simulink model "position_control"  (R2022a)
settings: Solver=ode1  StartTime=0.0  StopTime=inf  FixedStep=0.001  RelTol=1e-3
undefined symbols (not defined in the file or in its folder): a, b, k1, k2, kd2, kd4, kp2, kp4
libraries: arduinolib x19, arduinosensorlib x6, simulink_extras x2, visionfilter x1, eeLuenbergerObserver x1
settings Model: SimulationMode=external  ExtModeTrigDuration=2  Creator=DCLab  LastModifiedBy=LabPC
settings SolverCC: AllowMultiTaskInputOutput=on
settings OptimizationCC: EnhancedBackFolding=on  PassReuseOutputArgsAs=Individual arguments  ZeroExternalMemoryAtStartup=off  ZeroInternalMemoryAtStartup=off  MaxStackSize=64  OptimizeBlockOrder=speed  DifferentSizesBufferReuse=on  OptimizationCustomize=off  EfficientTunableParamExpr=on
settings DebuggingCC: ParameterTunabilityLossMsg=error  UnconnectedInputMsg=warning  UnconnectedOutputMsg=warning  UnconnectedLineMsg=warning
settings HardwareCC: ProdBitPerPointer=32  ProdBitPerSizeT=32  ProdBitPerPtrDiffT=32  ProdLargestAtomicInteger=Long  ProdLargestAtomicFloat=Double  ProdWordSize=32  ProdHWDeviceType=ARM Compatible->ARM Cortex
settings SFSimCC: MATLABDynamicMemAlloc=off  SimTargetLang=C++
settings RTWCC: SystemTargetFile=ert.tlc  HardwareBoard=Arduino Due  TemplateMakefile=ert_default_tmf  Toolchain=Arduino ARM  BuildConfiguration=Faster Runs  DLArmComputeVersion=19.05
settings CodeAppCC: ForceParamTrailComments=on  IgnoreCustomStorageClasses=off  OperatorAnnotations=on  SimulinkDataObjDesc=on  SFDataObjDesc=on  InsertBlockDesc=on
settings ERTTargetCC: SupportContinuousTime=on  SupportVariableSizeSignals=on  ExtMode=on  ExtModeTransport=3  ExtModeStaticAlloc=on  ExtModeStaticAllocSize=24576  ExtModeMexFile=ext_xcp  ExtModeMexArgs=0 3 115200  ExtModeIntrfLevel=Level2 - Open

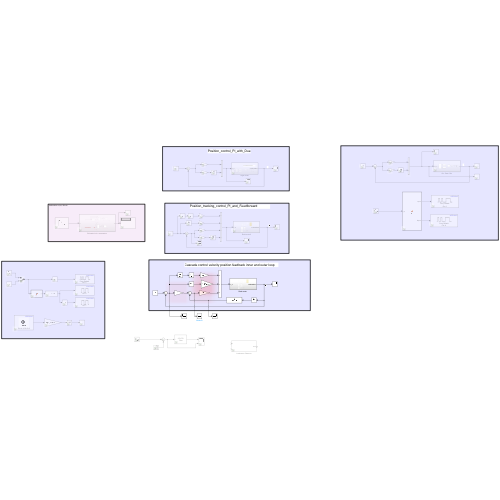
[thumbnail: Simulink's stored preview of the top-level diagram]
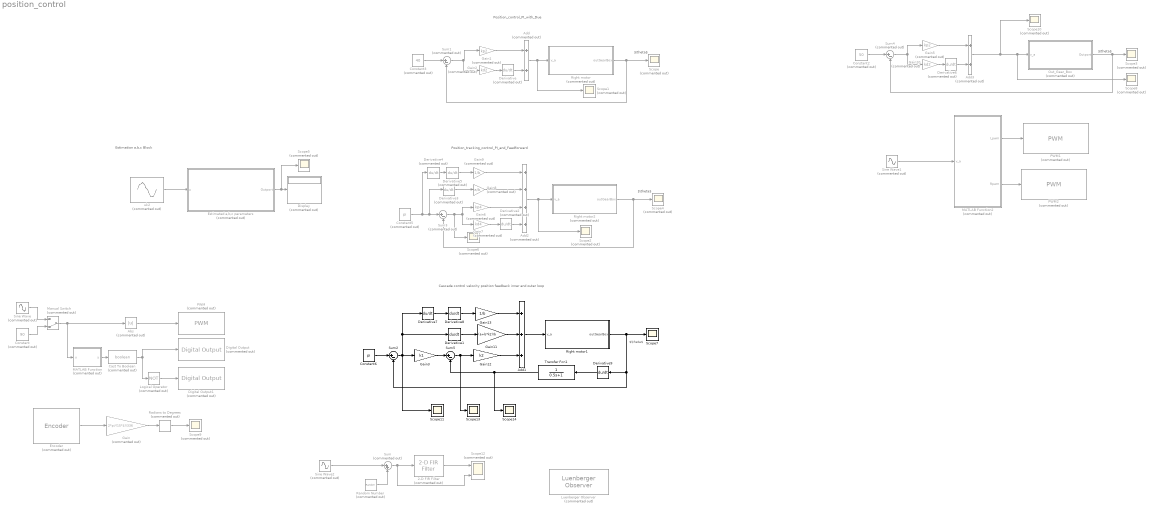
== system position_control ==
  note: Position_control_PI_with_Due
  note: $\theta$
  note: $\theta$
  note: Position_tracking_control_PI_and_Feedforward
  note: $\theta$
  note: Estimation a,b,c Block
  note: Cascade control velocity position feedback inner and outer loop
  note: $\theta$
  2-D FIR Filter : visionfilter/2-D FIR Filter  Commented=on  separable=off  filtSrc=Specify via dialog  filterMtrx=[1 0; 0 -1]  verticalFilter=[4 0]  horizontalFilter=[4 0]  outSize=Full  padType=Constant  padSrc=Specify via dialog  padVal=0  method=Convolution  firstCoeffMode=Specify word length  firstCoeffWordLength=16  firstCoeffFracLength=14  firstCoeffSignedness=Signed  firstCoeffLastDataTypeStr=fixdt(1,16)  outputSignedness=Auto  accumLastDataTypeStr=Inherit: Same as product output  prodOutputMode=Binary point scaling  prodOutputWordLength=32  prodOutputFracLength=10  prodOutputLastDataTypeStr=fixdt([],32,10)  roundingMode=Floor  overflowMode=off  firstCoeffDataTypeStr=fixdt(1,16)  firstCoeffMin=[]  firstCoeffMax=[]  prodOutputDataTypeStr=fixdt([],32,10)  accumDataTypeStr=Inherit: Same as product output  outputMin=[]  outputMax=[]
      settings: SourceProductBaseCode=VP
  Abs : Abs  Commented=on  SaturateOnIntegerOverflow=off
  Add : Sum  Commented=on
  Add1 : Sum  Inputs=+++
  Add2 : Sum  Commented=on  Inputs=++++
  Add3 : Sum  Commented=on
  Cast To Boolean : DataTypeConversion  Commented=on  OutDataTypeStr=boolean  SaturateOnIntegerOverflow=off  RndMeth=Floor
  Constant : Constant  Commented=on  Value=90
  Constant2 : Constant  Commented=on  Value=50
  Constant3 : Constant  Commented=on  Value=40
  Constant5 : Constant  Commented=on  Value=pi
  Constant6 : Constant  Value=pi
  Derivative{,2..6} (6 alike) : Derivative  Commented=on
  Derivative{1,7..9} (4 alike) : Derivative
  Digital Output : arduinolib/Digital Output  Commented=on  pinNumber=6  Direction=output  blockPlatform=arduino
  Digital Output1 : arduinolib/Digital Output  Commented=on  pinNumber=7  Direction=output  blockPlatform=arduino
  Display : Display  Commented=on
  Encoder : arduinosensorlib/Encoder  Commented=on  InputA=2  InputB=3  Mode=No reset  SampleTime=0.01
      settings: SourceProductBaseCode=ARDUINO
  Estimated a,b,c parameters : Subsystem  Commented=on
  Gain : Gain  Commented=on  Gain=2*pi/(15*4)/336
  Gain1 : Gain  Commented=on  Gain=kp2
  Gain10 : Gain  Commented=on  Gain=kd2
  Gain11 : Gain  Gain=(a+b*k2)/b
  Gain12 : Gain  Gain=k2
  Gain13 : Gain  Gain=1/b
  Gain2 : Gain  Commented=on  Gain=kd2
  Gain3 : Gain  Gain=k1
  Gain5 : Gain  Commented=on  Gain=kp2
  Gain6 : Gain  Commented=on  Gain=kp4
  Gain7 : Gain  Commented=on  Gain=kd4
  Gain8 : Gain  Commented=on  Gain=a/b
  Gain9 : Gain  Commented=on  Gain=1/b
  Logical Operator : Logic  Commented=on  Operator=NOT  AllPortsSameDT=off  OutDataTypeStr=boolean
  Luenberger Observer : eeLuenbergerObserver/Luenberger Observer  Commented=on  StateSpaceType=Discrete-time  Ad=1  Bd=1  Cd=1  Dd=1  A=1  B=1  C=1  D=1  ObserverDesign=Desired eigenvalues  Ld=1  DesiredEigenvalues=0  x0=0  Tsd=0.1  Ts=0.1
      settings: SourceProductBaseCode=PS
  MATLAB Function : MATLAB Function  Commented=on  TreatAsAtomicUnit=on
  MATLAB Function2 : MATLAB Function  Commented=on  TreatAsAtomicUnit=on
  Manual Switch : ManualSwitch  Commented=on  CurrentSetting=0
  Out_Gear_Box : Subsystem  Commented=on
  PWM : arduinolib/PWM  Commented=on  pinNumber=5  frequencyType=Default  desiredFrequency=490.2  achievableFrequency=490.2
  PWM1 : arduinolib/PWM  Commented=on  pinNumber=6  frequencyType=Default  desiredFrequency=490.2  achievableFrequency=490.2
  PWM2 : arduinolib/PWM  Commented=on  pinNumber=9  frequencyType=Default  desiredFrequency=490.2  achievableFrequency=490.2
  Radians to Degrees : simulink_extras/Transformations/Radians to Degrees  Commented=on
  Random Number : RandomNumber  Commented=on  Variance=0.001  SampleTime=0.01
  Right motor : Subsystem  Commented=on
  Right motor1 : Subsystem
  Right motor2 : Subsystem  Commented=on
  Scope{,1..6,8..10} (10 alike) : Scope  Commented=on
  Scope{7,11,13..14} (4 alike) : Scope
  Scope12 : Scope  Commented=on  NumInputPorts=2
  Sine Wave : Sin  Commented=on  Amplitude=2*pi  Frequency=2*pi*0.25  SampleTime=0
  Sine Wave1 : Sin  Commented=on  Amplitude=50  SampleTime=0
  Sine Wave2 : Sin  Commented=on  SampleTime=0.01
  Sum : Sum  Commented=on  Inputs=|++
  Sum1 : Sum  Commented=on  Inputs=|+-
  Sum2 : Sum  Inputs=|+-
  Sum3 : Sum  Commented=on  Inputs=|+-
  Sum4 : Sum  Commented=on  Inputs=|+-
  Sum5 : Sum  Inputs=|+-
  Transfer Fcn1 : TransferFcn  Denominator=[0.5 1]
  uk2 : Sin  Commented=on  Amplitude=12  Frequency=2*pi*1.2  SampleTime=0
  wires:
  Gain2/1 -> Derivative/1
  Sum1/1 -> Gain2/1, Gain1/1
  Derivative/1 -> Add/2
  Gain1/1 -> Add/1
  Add/1 -> Scope1/1, Right motor/1(v_a)
  Right motor/1(outGearBox) -> Sum1/2, Scope/1
  Constant3/1 -> Sum1/1
  Sum3/1 -> Scope6/1, Gain6/1, Gain7/1
  Gain9/1 -> Add2/1
  Derivative2/1 -> Add2/4
  Gain6/1 -> Add2/3
  Constant5/1 -> Derivative4/1, Derivative3/1, Sum3/1
  Gain7/1 -> Derivative2/1
  Gain8/1 -> Add2/2
  Derivative3/1 -> Gain8/1
  Derivative4/1 -> Derivative5/1
  Derivative5/1 -> Gain9/1
  Right motor2/1(outGearBox) -> Sum3/2, Scope4/1
  Add2/1 -> Scope2/1, Right motor2/1(v_a)
  MATLAB Function/1(y) -> Cast To Boolean/1
  Cast To Boolean/1 -> Logical Operator/1, Digital Output/1
  Logical Operator/1 -> Digital Output1/1
  Abs/1 -> PWM/1
  Encoder/1 -> Gain/1
  Sine Wave/1 -> Manual Switch/1
  Manual Switch/1 -> MATLAB Function/1(u), Abs/1
  Constant/1 -> Manual Switch/2
  Constant2/1 -> Sum4/1
  Add3/1 -> Out_Gear_Box/1(v_a), Scope8/1, Scope10/1
  Gain5/1 -> Add3/1
  Derivative6/1 -> Add3/2
  Sum4/1 -> Gain5/1, Gain10/1
  Gain10/1 -> Derivative6/1
  Gain/1 -> Radians to Degrees/1
  Radians to Degrees/1 -> Scope9/1
  Out_Gear_Box/1(Outport) -> Scope3/1, Sum4/2
  MATLAB Function2/1(Lpwm) -> PWM1/1
  MATLAB Function2/2(Rpwm) -> PWM2/1
  Sine Wave1/1 -> MATLAB Function2/1(v_a)
  Estimated a,b,c parameters/1(Outport) -> Scope5/1, Display/1
  uk2/1 -> Estimated a,b,c parameters/1(u)
  Gain12/1 -> Add1/3
  Derivative7/1 -> Derivative8/1
  Gain13/1 -> Add1/1
  Right motor1/1(outGearBox) -> Derivative9/1, Sum2/2, Scope7/1
  Sum2/1 -> Scope11/1, Derivative7/1, Derivative1/1, Gain3/1
  Sum5/1 -> Scope13/1, Gain12/1
  Gain11/1 -> Add1/2
  Gain3/1 -> Sum5/1
  Constant6/1 -> Sum2/1
  Derivative1/1 -> Gain11/1
  Derivative8/1 -> Gain13/1
  Add1/1 -> Right motor1/1(v_a)
  Random Number/1 -> Sum/2
  Sine Wave2/1 -> Sum/1
  Sum/1 -> Scope12/2, 2-D FIR Filter/1
  2-D FIR Filter/1 -> Scope12/1
  Derivative9/1 -> Transfer Fcn1/1
  Transfer Fcn1/1 -> Scope14/1, Sum5/2

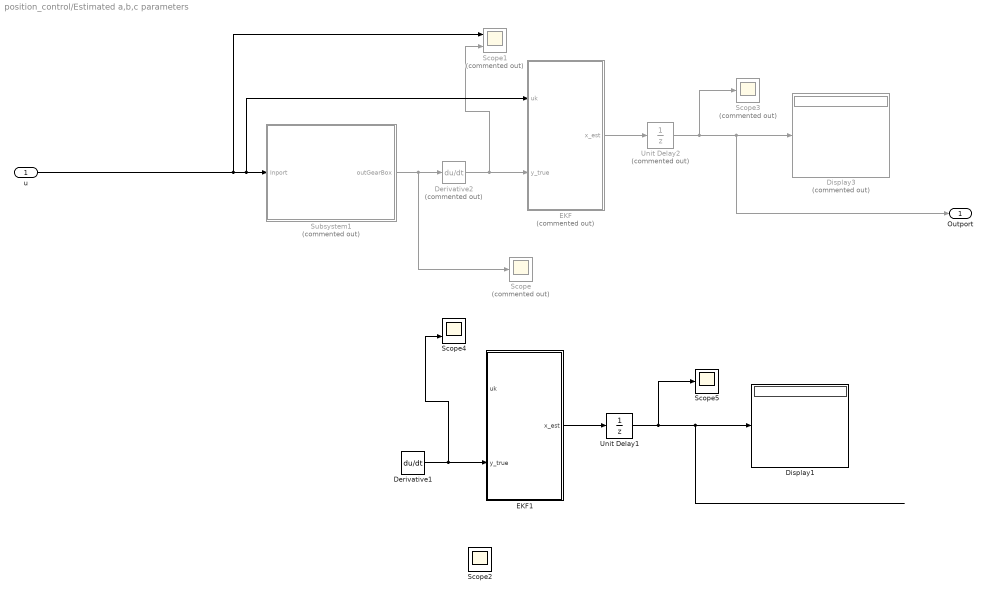
== system position_control/Estimated a,b,c parameters ==
  u : Inport
  Derivative1 : Derivative
  Derivative2 : Derivative  Commented=on
  Display1 : Display
  Display3 : Display  Commented=on
  EKF : MATLAB Function  Commented=on  TreatAsAtomicUnit=on
  EKF1 : MATLAB Function  TreatAsAtomicUnit=on
  Scope : Scope  Commented=on
  Scope1 : Scope  Commented=on  NumInputPorts=2
  Scope2 : Scope
  Scope3 : Scope  Commented=on
  Scope4 : Scope  NumInputPorts=2
  Scope5 : Scope
  Subsystem1 : Subsystem  Commented=on
  Unit Delay1 : UnitDelay  InitialCondition=[0;0;0;0]  SampleTime=-1  HasFrameUpgradeWarning=on
  Unit Delay2 : UnitDelay  Commented=on  InitialCondition=[0;0;0;0]  SampleTime=-1  HasFrameUpgradeWarning=on
  Outport : Outport
  wires:
  Derivative2/1 -> Scope1/2, EKF/2(y_true)
  Unit Delay2/1 -> Outport/1, Display3/1, Scope3/1
  EKF/1(x_est) -> Unit Delay2/1
  Subsystem1/1(outGearBox) -> Scope/1, Derivative2/1
  u/1 -> Scope1/1, Subsystem1/1(Inport), EKF/1(uk)
  ? -> ?
  ? -> Derivative1/1, Scope2/1
  EKF1/1(x_est) -> Unit Delay1/1
  Unit Delay1/1 -> Scope5/1, Display1/1
  Derivative1/1 -> EKF1/2(y_true), Scope4/2

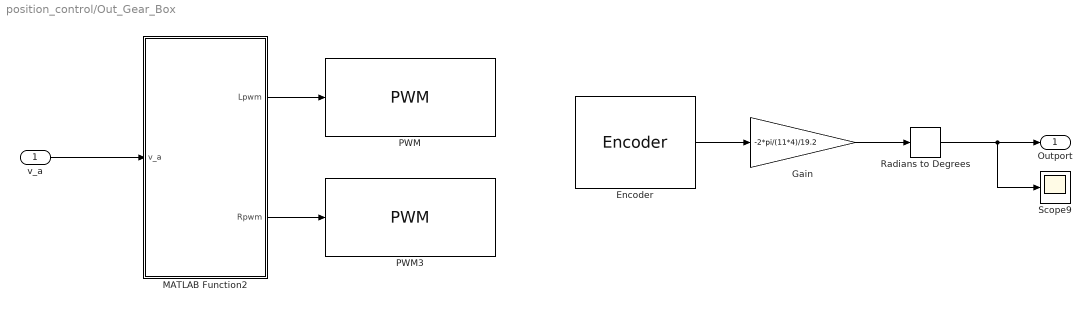
== system position_control/Out_Gear_Box ==
  v_a : Inport
  Encoder : arduinosensorlib/Encoder  InputA=2  InputB=3  Mode=No reset  SampleTime=0.01
      settings: SourceProductBaseCode=ARDUINO
  Gain : Gain  Gain=-2*pi/(11*4)/19.2
  MATLAB Function2 : MATLAB Function  TreatAsAtomicUnit=on
  PWM : arduinolib/PWM  pinNumber=6  frequencyType=Default  desiredFrequency=490.2  achievableFrequency=490.2
  PWM3 : arduinolib/PWM  pinNumber=7  frequencyType=Default  desiredFrequency=490.2  achievableFrequency=490.2
  Radians to Degrees : simulink_extras/Transformations/Radians to Degrees
  Scope9 : Scope
  Outport : Outport
  wires:
  MATLAB Function2/1(Lpwm) -> PWM/1
  v_a/1 -> MATLAB Function2/1(v_a)
  Gain/1 -> Radians to Degrees/1
  Encoder/1 -> Gain/1
  Radians to Degrees/1 -> Outport/1, Scope9/1
  MATLAB Function2/2(Rpwm) -> PWM3/1

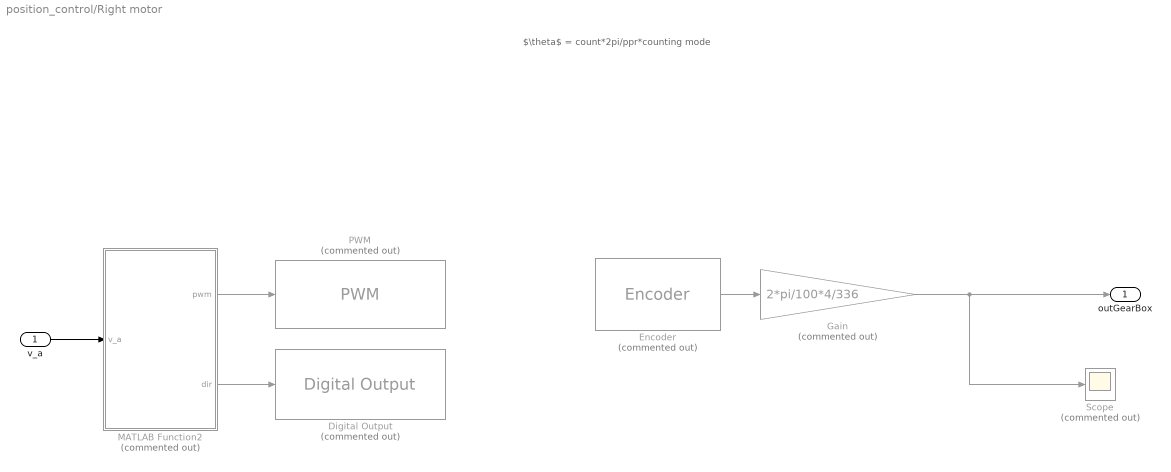
== system position_control/Right motor ==
  note: $\theta$ = count*2pi/ppr*counting mode
  v_a : Inport
  Digital Output : arduinolib/Digital Output  Commented=on  pinNumber=7  Direction=output  blockPlatform=arduino
  Encoder : arduinosensorlib/Encoder  Commented=on  InputA=2  InputB=3  Mode=No reset  SampleTime=-1
      settings: SourceProductBaseCode=ARDUINO
  Gain : Gain  Commented=on  Gain=2*pi/100*4/336
  MATLAB Function2 : MATLAB Function  Commented=on  TreatAsAtomicUnit=on
  PWM : arduinolib/PWM  Commented=on  pinNumber=6  frequencyType=Default  desiredFrequency=490.2  achievableFrequency=490.2
  Scope : Scope  Commented=on
  outGearBox : Outport
  wires:
  v_a/1 -> MATLAB Function2/1(v_a)
  MATLAB Function2/2(dir) -> Digital Output/1
  MATLAB Function2/1(pwm) -> PWM/1
  Encoder/1 -> Gain/1
  Gain/1 -> Scope/1, outGearBox/1

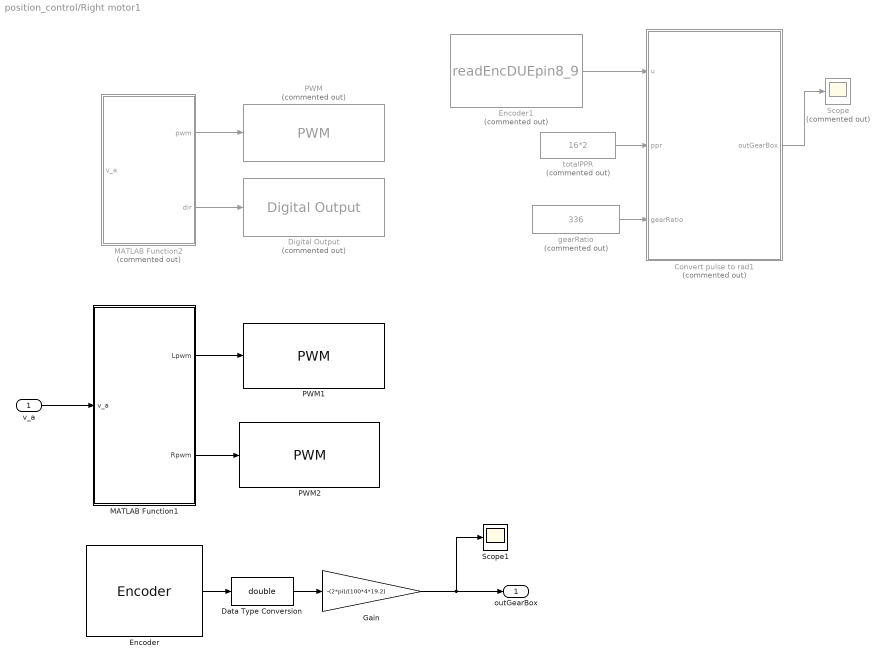
== system position_control/Right motor1 ==
  v_a : Inport
  Convert pulse to rad1 : MATLAB Function  Commented=on  TreatAsAtomicUnit=on
  Data Type Conversion : DataTypeConversion  OutDataTypeStr=double  SaturateOnIntegerOverflow=off  RndMeth=Floor
  Digital Output : arduinolib/Digital Output  Commented=on  pinNumber=7  Direction=output  blockPlatform=arduino
  Encoder : arduinosensorlib/Encoder  InputA=2  InputB=3  Mode=No reset  SampleTime=0.01
      settings: SourceProductBaseCode=ARDUINO
  Encoder1 : S-Function  Commented=on  InitFcn=try, set_param(gcb,'FunctionName','readEncDUEpin8_9'), end  FunctionName=readEncDUEpin8_9  SFunctionModules=readEncDUEpin8_9_wrapper  SFunctionDeploymentMode=off  EnableBusSupport=off  mask(S-Function Builder){}
      mask help: Simulink:masks:SFunctionBuilder_MD
      mask init:
      | val = [[.9  0.75 0.75 1 1 .9 .9 1]',[1 1 0.75 0.75 .9 .9 1 .9]'];try , sys = get_param(gcb,'SfunBuilderFcnName');if isempty(sys), sys = get_param(gcb,'FunctionName'); end,catch, sys = get_param(gcb,'FunctionName'); end
      settings: CopyFcn=set_param(gcbh,'LinkStatus','none')  PreSaveFcn=try, set_param(gcb,'FunctionName','readEncDUEpin8_9'), end  OpenFcn=sfunctionwizard(gcbh)
      mask Display:
      | plot(val(:,1),val(:,2))
      | disp(sys)
      | port_label('output',1,'count')
  Gain : Gain  Gain=-(2*pi)/(100*4*19.2)
  MATLAB Function1 : MATLAB Function  TreatAsAtomicUnit=on
  MATLAB Function2 : MATLAB Function  Commented=on  TreatAsAtomicUnit=on
  PWM : arduinolib/PWM  Commented=on  pinNumber=5  frequencyType=Default  desiredFrequency=490.2  achievableFrequency=490.2
  PWM1 : arduinolib/PWM  pinNumber=6  frequencyType=Default  desiredFrequency=490.2  achievableFrequency=490.2
  PWM2 : arduinolib/PWM  pinNumber=7  frequencyType=Default  desiredFrequency=490.2  achievableFrequency=490.2
  Scope : Scope  Commented=on
  Scope1 : Scope
  gearRatio : Constant  Commented=on  Value=336
  totalPPR : Constant  Commented=on  Value=16*2
  outGearBox : Outport
  wires:
  Gain/1 -> Scope1/1, outGearBox/1
  Encoder/1 -> Data Type Conversion/1
  v_a/1 -> MATLAB Function1/1(v_a)
  MATLAB Function1/2(Rpwm) -> PWM2/1
  MATLAB Function1/1(Lpwm) -> PWM1/1
  Encoder1/1 -> Convert pulse to rad1/1(u)
  Convert pulse to rad1/1(outGearBox) -> Scope/1
  gearRatio/1 -> Convert pulse to rad1/3(gearRatio)
  MATLAB Function2/1(pwm) -> PWM/1
  MATLAB Function2/2(dir) -> Digital Output/1
  totalPPR/1 -> Convert pulse to rad1/2(ppr)
  Data Type Conversion/1 -> Gain/1

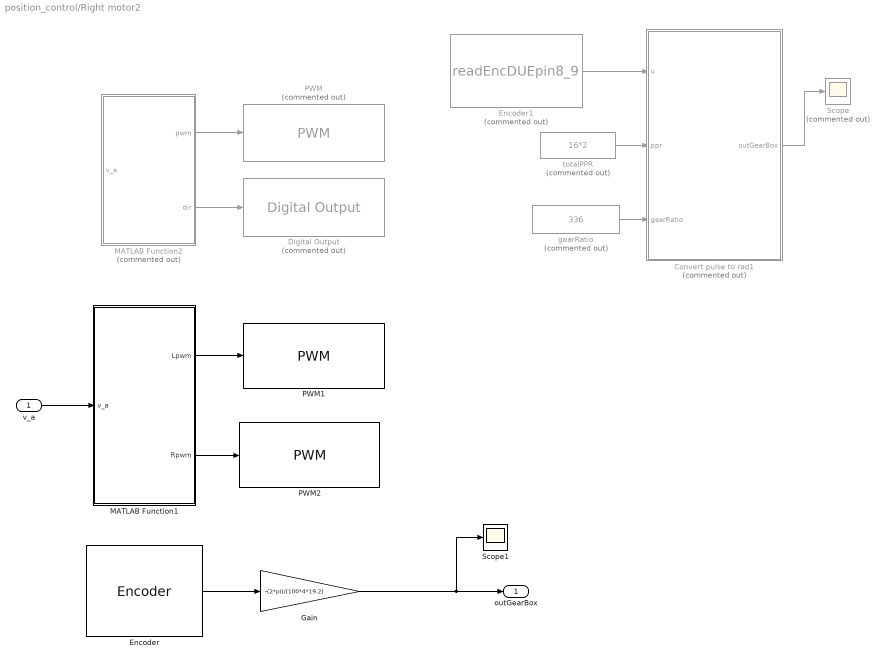
== system position_control/Right motor2 ==
  v_a : Inport
  Convert pulse to rad1 : MATLAB Function  Commented=on  TreatAsAtomicUnit=on
  Digital Output : arduinolib/Digital Output  Commented=on  pinNumber=7  Direction=output  blockPlatform=arduino
  Encoder : arduinosensorlib/Encoder  InputA=2  InputB=3  Mode=No reset  SampleTime=0.01
      settings: SourceProductBaseCode=ARDUINO
  Encoder1 : S-Function  Commented=on  InitFcn=try, set_param(gcb,'FunctionName','readEncDUEpin8_9'), end  FunctionName=readEncDUEpin8_9  SFunctionModules=readEncDUEpin8_9_wrapper  SFunctionDeploymentMode=off  EnableBusSupport=off  mask(S-Function Builder){}
      mask help: Simulink:masks:SFunctionBuilder_MD
      mask init: same as position_control/Right motor1/Encoder1
      settings: CopyFcn=set_param(gcbh,'LinkStatus','none')  PreSaveFcn=try, set_param(gcb,'FunctionName','readEncDUEpin8_9'), end  OpenFcn=sfunctionwizard(gcbh)
      mask Display:
      | plot(val(:,1),val(:,2))
      | disp(sys)
      | port_label('output',1,'count')
  Gain : Gain  Gain=-(2*pi)/(100*4*19.2)
  MATLAB Function1 : MATLAB Function  TreatAsAtomicUnit=on
  MATLAB Function2 : MATLAB Function  Commented=on  TreatAsAtomicUnit=on
  PWM : arduinolib/PWM  Commented=on  pinNumber=5  frequencyType=Default  desiredFrequency=490.2  achievableFrequency=490.2
  PWM1 : arduinolib/PWM  pinNumber=6  frequencyType=Default  desiredFrequency=490.2  achievableFrequency=490.2
  PWM2 : arduinolib/PWM  pinNumber=7  frequencyType=Default  desiredFrequency=490.2  achievableFrequency=490.2
  Scope : Scope  Commented=on
  Scope1 : Scope
  gearRatio : Constant  Commented=on  Value=336
  totalPPR : Constant  Commented=on  Value=16*2
  outGearBox : Outport
  wires:
  totalPPR/1 -> Convert pulse to rad1/2(ppr)
  MATLAB Function2/2(dir) -> Digital Output/1
  MATLAB Function2/1(pwm) -> PWM/1
  gearRatio/1 -> Convert pulse to rad1/3(gearRatio)
  Convert pulse to rad1/1(outGearBox) -> Scope/1
  Encoder1/1 -> Convert pulse to rad1/1(u)
  MATLAB Function1/1(Lpwm) -> PWM1/1
  MATLAB Function1/2(Rpwm) -> PWM2/1
  v_a/1 -> MATLAB Function1/1(v_a)
  Encoder/1 -> Gain/1
  Gain/1 -> Scope1/1, outGearBox/1

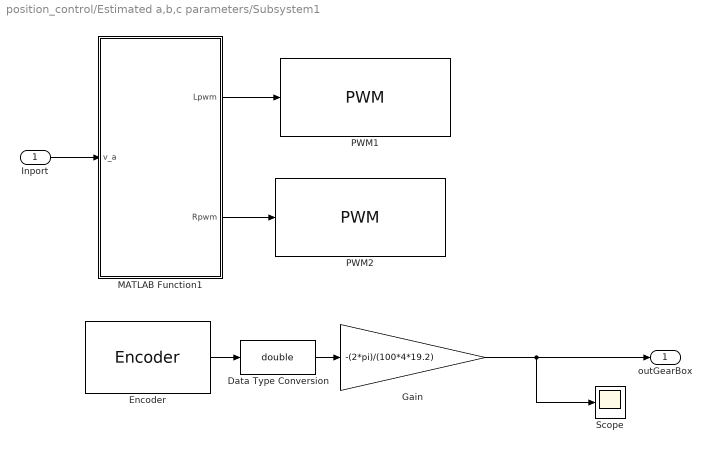
== system position_control/Estimated a,b,c parameters/Subsystem1 ==
  Inport : Inport
  Data Type Conversion : DataTypeConversion  OutDataTypeStr=double  SaturateOnIntegerOverflow=off  RndMeth=Floor
  Encoder : arduinosensorlib/Encoder  InputA=2  InputB=3  Mode=No reset  SampleTime=-1
      settings: SourceProductBaseCode=ARDUINO
  Gain : Gain  Gain=-(2*pi)/(100*4*19.2)
  MATLAB Function1 : MATLAB Function  TreatAsAtomicUnit=on
  PWM1 : arduinolib/PWM  pinNumber=6  frequencyType=Default  desiredFrequency=490.2  achievableFrequency=490.2
  PWM2 : arduinolib/PWM  pinNumber=7  frequencyType=Default  desiredFrequency=490.2  achievableFrequency=490.2
  Scope : Scope
  outGearBox : Outport
  wires:
  Gain/1 -> Scope/1, outGearBox/1
  Encoder/1 -> Data Type Conversion/1
  Data Type Conversion/1 -> Gain/1
  MATLAB Function1/1(Lpwm) -> PWM1/1
  MATLAB Function1/2(Rpwm) -> PWM2/1
  Inport/1 -> MATLAB Function1/1(v_a)

== matlab function position_control/Right motor1/MATLAB Function2 ==
  data: v_a input; pwm output; dir output
function [pwm,dir] = fcn(v_a)

vmax = 22.9;
%vmax = 10;
pwm_cal = v_a*254/vmax;
if pwm_cal > 0
    pwm = pwm_cal;
    dir = 0;
elseif pwm_cal < 0
    pwm = abs(pwm_cal);
    dir = 1;
else
    pwm = 0;
    dir = 0;
end

== matlab function position_control/Estimated a,b,c parameters/EKF1 ==
  settings: updateMethod=DISCRETE
  data: uk input; y_true input; x_est output
function x_est = fcn(uk,y_true)
Ts=0.01;
persistent x_est_p P Qd_est R_est Qc_est;
if isempty(x_est_p)
          
          x_est_p=[2;16;3.5;2];
          P=2*eye(4);
         Qc_est=1e-3*diag([10,10,10,1]);
          Qd_est=Qc_est*Ts;
          R_est=0.02;
end
c=[1 0 0 0];D=0;Ck=c;Dk=D;
%Comput Kalman Gain and update predicted value
Wk=P*Ck'/(Ck*P*Ck'+R_est);
y_est=Ck*x_est_p+Dk*uk;
x=x_est_p+Wk.*(y_true-y_est);
%Compute prediction at next time step
x_est=x+Ts*[-x(2)*x(1)+uk*x(3)-x(4)*sign(x(1));0;0;0];
%Update error covariance matrices
P=P-Wk*Ck*P;
%Define Ak
Ak=eye(4)+Ts*[-x(2) -x(1) uk -sign(x(1));0 0 0 0;0 0 0 0;0 0 0 0];
P=Ak*P*Ak'+Qd_est;
x_est_p=x_est;

== matlab function position_control/MATLAB Function2 ==
  data: v_a input; Lpwm output; Rpwm output
function [Lpwm,Rpwm] = fcn(v_a)

vmax = 22.9;
pwm_cal = v_a*254/vmax;

if pwm_cal > 0
    Lpwm = 0;
    Rpwm = pwm_cal;
elseif pwm_cal < 0
    Lpwm = abs(pwm_cal);
    Rpwm = 0;
else
    Lpwm = 0;
    Rpwm = 0;
end

== matlab function position_control/MATLAB Function ==
  data: u input; y output
function y = fcn(u)

y = (sign(u)+1)/2;

== matlab function position_control/Right motor2/Convert pulse to rad1 ==
  settings: updateMethod=DISCRETE
  data: u input; ppr input; gearRatio input; outGearBox output
function outGearBox = fcn(u,ppr,gearRatio)

persistent counter_num over_flag
if(isempty(counter_num)), counter_num = 0;end
if(isempty(over_flag)), over_flag = 0;end
pulse2radian = 2*pi/ppr; % 1 pulse = ?? radian

if(double(u) - counter_num > 40000), over_flag = over_flag-1;
elseif(double(u) - counter_num < -40000), over_flag = over_flag+1;
end

inGearBox = (double(u)+over_flag*(2^32 -1))*pulse2radian; 
outGearBox = inGearBox/gearRatio;
counter_num = double(u) ;

== matlab function position_control/Right motor2/MATLAB Function2 ==
  data: v_a input; pwm output; dir output
function [pwm,dir] = fcn(v_a)

vmax = 22.9;
%vmax = 10;
pwm_cal = v_a*254/vmax;
if pwm_cal > 0
    pwm = pwm_cal;
    dir = 0;
elseif pwm_cal < 0
    pwm = abs(pwm_cal);
    dir = 1;
else
    pwm = 0;
    dir = 0;
end

== matlab function position_control/Out_Gear_Box/MATLAB Function2 ==
  data: v_a input; Lpwm output; Rpwm output
function [Lpwm,Rpwm] = fcn(v_a)

vmax = 22.9;
pwm_cal = v_a*254/vmax;

if pwm_cal > 0
    Lpwm = 0;
    Rpwm = pwm_cal;
elseif pwm_cal < 0
    Lpwm = abs(pwm_cal);
    Rpwm = 0;
else
    Lpwm = 0;
    Rpwm = 0;
end

== matlab function position_control/Right motor/MATLAB Function2 ==
  data: v_a input; pwm output; dir output
function [pwm,dir] = fcn(v_a)

vmax = 22.9;
pwm_cal = v_a*254/vmax;
if pwm_cal > 0
    pwm = pwm_cal;
    dir = 0;
elseif pwm_cal < 0
    pwm = abs(pwm_cal);
    dir = 1;
else
    pwm = 0;
    dir = 0;
end

== matlab function position_control/Right motor2/MATLAB Function1 ==
  data: v_a input; Lpwm output; Rpwm output
function [Lpwm,Rpwm] = fcn(v_a)

vmax = 22.9;
pwm_cal = v_a*254/vmax;

if pwm_cal > 0
    Lpwm = 0;
    Rpwm = pwm_cal;
elseif pwm_cal < 0
    Lpwm = abs(pwm_cal);
    Rpwm = 0;
else
    Lpwm = 0;
    Rpwm = 0;
end

== matlab function position_control/Estimated a,b,c parameters/EKF ==
  settings: updateMethod=DISCRETE
  data: uk input; y_true input; x_est output
function x_est = fcn(uk,y_true)
Ts=0.01;
persistent x_est_p P Qd_est R_est Qc_est;
if isempty(x_est_p)
          
          x_est_p=[2;16;3.5;2];
          P=2*eye(4);
         Qc_est=1e-3*diag([10,10,10,1]);
          Qd_est=Qc_est*Ts;
          R_est=0.02;
end
c=[1 0 0 0];D=0;Ck=c;Dk=D;
%Comput Kalman Gain and update predicted value
Wk=P*Ck'/(Ck*P*Ck'+R_est);
y_est=Ck*x_est_p+Dk*uk;
x=x_est_p+Wk.*(y_true-y_est);
%Compute prediction at next time step
x_est=x+Ts*[-x(2)*x(1)+uk*x(3)-x(4)*sign(x(1));0;0;0];
%Update error covariance matrices
P=P-Wk*Ck*P;
%Define Ak
Ak=eye(4)+Ts*[-x(2) -x(1) uk -sign(x(1));0 0 0 0;0 0 0 0;0 0 0 0];
P=Ak*P*Ak'+Qd_est;
x_est_p=x_est;

== matlab function position_control/Estimated a,b,c parameters/Subsystem1/MATLAB Function1 ==
  data: v_a input; Lpwm output; Rpwm output
function [Lpwm,Rpwm] = fcn(v_a)

vmax = 22.9;
pwm_cal = v_a*254/vmax;

if pwm_cal > 0
    Lpwm = 0;
    Rpwm = pwm_cal;
elseif pwm_cal < 0
    Lpwm = abs(pwm_cal);
    Rpwm = 0;
else
    Lpwm = 0;
    Rpwm = 0;
end

== matlab function position_control/Right motor1/Convert pulse to rad1 ==
  settings: updateMethod=DISCRETE
  data: u input; ppr input; gearRatio input; outGearBox output
function outGearBox = fcn(u,ppr,gearRatio)

persistent counter_num over_flag
if(isempty(counter_num)), counter_num = 0;end
if(isempty(over_flag)), over_flag = 0;end
pulse2radian = 2*pi/ppr; % 1 pulse = ?? radian

if(double(u) - counter_num > 40000), over_flag = over_flag-1;
elseif(double(u) - counter_num < -40000), over_flag = over_flag+1;
end

inGearBox = (double(u)+over_flag*(2^32 -1))*pulse2radian; 
outGearBox = inGearBox/gearRatio;
counter_num = double(u) ;

== matlab function position_control/Right motor1/MATLAB Function1 ==
  data: v_a input; Lpwm output; Rpwm output
function [Lpwm,Rpwm] = fcn(v_a)

vmax = 22.9;
pwm_cal = v_a*254/vmax;

if pwm_cal > 0
    Lpwm = 0;
    Rpwm = pwm_cal;
elseif pwm_cal < 0
    Lpwm = abs(pwm_cal);
    Rpwm = 0;
else
    Lpwm = 0;
    Rpwm = 0;
end
